simulink model "lab3_5_6"  (R2018a)
settings: Solver=VariableStepAuto  StartTime=0.0  StopTime=Tsim*Ts  RelTol=1e-3
values from neighbouring files (symbols this model uses):
  alpha = 0.99    [lab3.m]
  c_ik_init = zeros(26,1)    [lab3.m]
  coefHybrid = [0 0.2 1 0.3 -0.4 -0.1 0.1 -0.05 -0.02 -0.01]    [lab3.m]
  G = 0.1    [lab3.m]
  mu = mu_try(i)    [lab3.m]
  scramblerLocal = [3 5]    [lab3.m]
  scramblerRemote = [5 7]    [lab3.m]
  Ts = 1    [lab3.m]
settings Model: Creator=leonardopedroso  LastModifiedBy=leonardopedroso

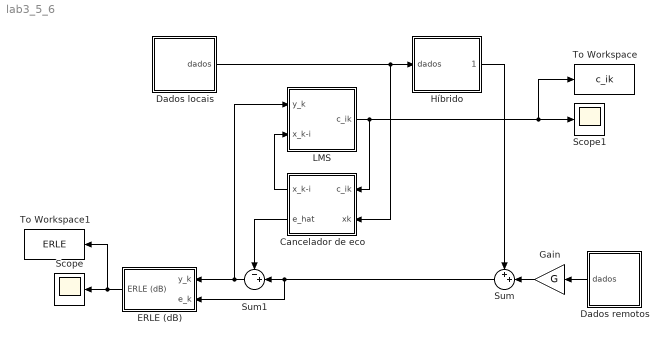
== system lab3_5_6 ==
  "Cancelador de eco " : Subsystem
  Dados locais : Subsystem
  Dados remotos : Subsystem
  ERLE (dB) : Subsystem
  Gain : Gain  Gain=G
  Híbrido : Subsystem
  LMS : Subsystem
  Scope : Scope
  Scope1 : Scope
  Sum : Sum  Inputs=++|
  Sum1 : Sum  Inputs=-+|
  To Workspace : ToWorkspace  VariableName=c_ik  SaveFormat=Timeseries  SampleTime=-1
  To Workspace1 : ToWorkspace  VariableName=ERLE  SaveFormat=Timeseries  SampleTime=-1
  wires:
  Dados locais/1(dados) -> Híbrido/1(dados), "Cancelador de eco "/2("xk ")
  Híbrido/1(híbrido) -> Sum/1
  Gain/1 -> Sum/2
  Dados remotos/1(dados) -> Gain/1
  Sum/1 -> Sum1/2, ERLE (dB)/2(e_k)
  LMS/1(c_ik) -> "Cancelador de eco "/1(c_ik), Scope1/1, To Workspace/1
  Sum1/1 -> ERLE (dB)/1(y_k), LMS/1("y_k ")
  "Cancelador de eco "/2("e_hat ") -> Sum1/1
  "Cancelador de eco "/1(x_k-i) -> LMS/2(x_k-i)
  ERLE (dB)/1(ERLE (dB)) -> To Workspace1/1, Scope/1

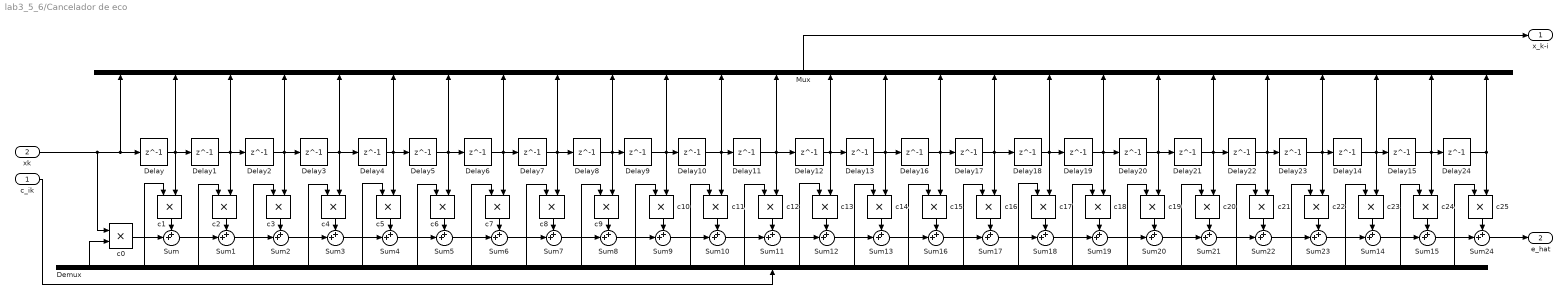
== system lab3_5_6/Cancelador de eco  ==
  c_ik : Inport
  "xk " : Inport  Port=2
  Delay{,1..24} (25 alike) : Delay  DelayLength=1  SampleTime=Ts
  Demux : Demux  Outputs=26
  Mux : Mux  Inputs=26
  Sum{,1..24} (25 alike) : Sum  Inputs=++|
  c{0..25} (26 alike) : Product
  x_k-i : Outport
  "e_hat " : Outport  Port=2
  wires:
  "xk "/1 -> Delay/1, Mux/1, c0/1
  Delay/1 -> Delay1/1, Mux/2, c1/2
  Delay1/1 -> Delay2/1, Mux/3, c2/2
  Delay2/1 -> Mux/4, Delay3/1, c3/2
  c1/1 -> Sum/1
  c0/1 -> Sum/2
  c3/1 -> Sum2/1
  c2/1 -> Sum1/1
  c4/1 -> Sum3/1
  Sum/1 -> Sum1/2
  Sum1/1 -> Sum2/2
  Sum2/1 -> Sum3/2
  c_ik/1 -> Demux/1
  Demux/5 -> c4/1
  Demux/4 -> c3/1
  Demux/3 -> c2/1
  Demux/2 -> c1/1
  Demux/1 -> c0/2
  c7/1 -> Sum6/1
  Delay5/1 -> Delay6/1, Mux/7, c6/2
  Delay4/1 -> Delay5/1, Mux/6, c5/2
  c8/1 -> Sum7/1
  Sum5/1 -> Sum6/2
  Sum4/1 -> Sum5/2
  Sum6/1 -> Sum7/2
  c6/1 -> Sum5/1
  Demux/8 -> c7/1
  Sum3/1 -> Sum4/2
  c5/1 -> Sum4/1
  Demux/6 -> c5/1
  Demux/7 -> c6/1
  Demux/9 -> c8/1
  Delay6/1 -> Mux/8, Delay7/1, c7/2
  Delay3/1 -> Mux/5, Delay4/1, c4/2
  c11/1 -> Sum10/1
  Delay9/1 -> c10/2, Mux/11, Delay10/1
  Delay8/1 -> c9/2, Mux/10, Delay9/1
  c12/1 -> Sum11/1
  Sum9/1 -> Sum10/2
  Sum8/1 -> Sum9/2
  Sum10/1 -> Sum11/2
  c10/1 -> Sum9/1
  Demux/12 -> c11/1
  Sum7/1 -> Sum8/2
  c9/1 -> Sum8/1
  Demux/10 -> c9/1
  Demux/11 -> c10/1
  Demux/13 -> c12/1
  Delay10/1 -> c11/2, Delay11/1, Mux/12
  Delay7/1 -> Mux/9, Delay8/1, c8/2
  Sum21/1 -> Sum22/2
  Demux/19 -> c18/1
  Delay12/1 -> Mux/14, Delay13/1, c13/2
  c15/1 -> Sum16/1
  c24/1 -> Sum15/1
  Demux/25 -> c24/1
  Demux/22 -> c21/1
  Demux/23 -> c22/1
  Sum16/1 -> Sum17/2
  Delay22/1 -> Mux/22, c21/2, Delay23/1
  c21/1 -> Sum22/1
  Demux/20 -> c19/1
  c22/1 -> Sum23/1
  c16/1 -> Sum17/1
  Delay13/1 -> Mux/15, Delay16/1, c14/2
  c18/1 -> Sum19/1
  Sum13/1 -> Sum16/2
  Sum12/1 -> Sum13/2
  Demux/15 -> c14/1
  Delay17/1 -> Mux/17, Delay18/1, c16/2
  Delay11/1 -> Delay12/1, Mux/13, c12/2
  Demux/16 -> c15/1
  Sum11/1 -> Sum12/2
  c14/1 -> Sum13/1
  c13/1 -> Sum12/1
  Demux/17 -> c16/1
  Demux/14 -> c13/1
  Demux/24 -> c23/1
  Sum22/1 -> Sum23/2
  Sum17/1 -> Sum18/2
  Delay16/1 -> Mux/16, Delay17/1, c15/2
  Demux/18 -> c17/1
  Delay18/1 -> Mux/18, Delay19/1, c17/2
  c19/1 -> Sum20/1
  Demux/21 -> c20/1
  Delay20/1 -> Mux/20, Delay21/1, c19/2
  Delay19/1 -> Mux/19, Delay20/1, c18/2
  Sum19/1 -> Sum20/2
  c20/1 -> Sum21/1
  c17/1 -> Sum18/1
  Sum18/1 -> Sum19/2
  Sum20/1 -> Sum21/2
  Delay21/1 -> Mux/21, Delay22/1, c20/2
  Sum14/1 -> Sum15/2
  Sum23/1 -> Sum14/2
  Delay23/1 -> Mux/23, c22/2, Delay14/1
  c23/1 -> Sum14/1
  Delay14/1 -> Mux/24, c23/2, Delay15/1
  Delay15/1 -> Delay24/1, Mux/25, c24/2
  Delay24/1 -> Mux/26, c25/2
  Sum15/1 -> Sum24/2
  c25/1 -> Sum24/1
  Demux/26 -> c25/1
  Sum24/1 -> "e_hat "/1
  Mux/1 -> x_k-i/1

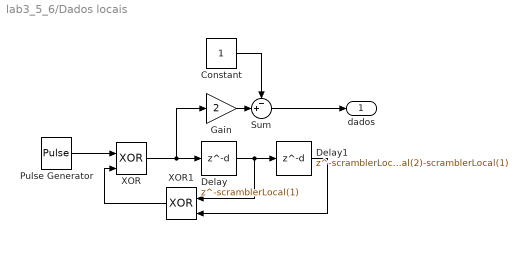
== system lab3_5_6/Dados locais ==
  Constant : Constant
  Delay : Delay  DelayLength=scramblerLocal(1)  SampleTime=Ts
  Delay1 : Delay  DelayLength=scramblerLocal(2)-scramblerLocal(1)  SampleTime=Ts
  Gain : Gain  Gain=2
  Pulse Generator : DiscretePulseGenerator  PulseType=Time based  Period=2*Ts  PulseWidth=50
  Sum : Sum  Inputs=-+|
  XOR : Logic  Operator=XOR  IconShape=distinctive  AllPortsSameDT=off  OutDataTypeStr=boolean
  XOR1 : Logic  Operator=XOR  IconShape=distinctive  AllPortsSameDT=off  OutDataTypeStr=boolean
  dados : Outport
  wires:
  Pulse Generator/1 -> XOR/1
  XOR1/1 -> XOR/2
  Delay/1 -> XOR1/1, Delay1/1
  Delay1/1 -> XOR1/2
  Gain/1 -> Sum/2
  Constant/1 -> Sum/1
  XOR/1 -> Delay/1, Gain/1
  Sum/1 -> dados/1

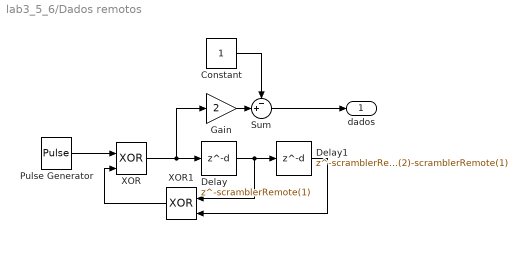
== system lab3_5_6/Dados remotos ==
  Constant : Constant
  Delay : Delay  DelayLength=scramblerRemote(1)  SampleTime=Ts
  Delay1 : Delay  DelayLength=scramblerRemote(2)-scramblerRemote(1)  SampleTime=Ts
  Gain : Gain  Gain=2
  Pulse Generator : DiscretePulseGenerator  PulseType=Time based  Period=2*Ts  PulseWidth=50
  Sum : Sum  Inputs=-+|
  XOR : Logic  Operator=XOR  IconShape=distinctive  AllPortsSameDT=off  OutDataTypeStr=boolean
  XOR1 : Logic  Operator=XOR  IconShape=distinctive  AllPortsSameDT=off  OutDataTypeStr=boolean
  dados : Outport
  wires:
  Pulse Generator/1 -> XOR/1
  XOR1/1 -> XOR/2
  Delay/1 -> XOR1/1, Delay1/1
  Delay1/1 -> XOR1/2
  Gain/1 -> Sum/2
  Constant/1 -> Sum/1
  XOR/1 -> Delay/1, Gain/1
  Sum/1 -> dados/1

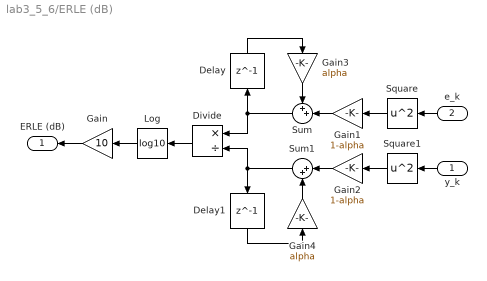
== system lab3_5_6/ERLE (dB) ==
  y_k : Inport
  e_k : Inport  Port=2
  Delay : Delay  DelayLength=1  SampleTime=Ts
  Delay1 : Delay  DelayLength=1  SampleTime=Ts
  Divide : Product  Inputs=*/
  Gain : Gain  Gain=10
  Gain1 : Gain  Gain=1-alpha
  Gain2 : Gain  Gain=1-alpha
  Gain3 : Gain  Gain=alpha
  Gain4 : Gain  Gain=alpha
  Log : Math  Operator=log10  SaturateOnIntegerOverflow=on
  Square : Math  Operator=square  SaturateOnIntegerOverflow=on
  Square1 : Math  Operator=square  SaturateOnIntegerOverflow=on
  Sum : Sum  Inputs=++|
  Sum1 : Sum  Inputs=|++
  ERLE (dB) : Outport
  wires:
  Gain/1 -> ERLE (dB)/1
  Log/1 -> Gain/1
  Divide/1 -> Log/1
  e_k/1 -> Square/1
  y_k/1 -> Square1/1
  Square/1 -> Gain1/1
  Square1/1 -> Gain2/1
  Gain1/1 -> Sum/2
  Sum/1 -> Divide/1, Delay/1
  Delay/1 -> Gain3/1
  Gain3/1 -> Sum/1
  Delay1/1 -> Gain4/1
  Sum1/1 -> Divide/2, Delay1/1
  Gain2/1 -> Sum1/1
  Gain4/1 -> Sum1/2

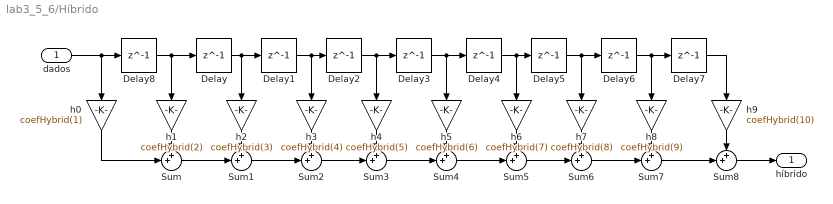
== system lab3_5_6/Híbrido ==
  dados : Inport
  Delay{,1..8} (9 alike) : Delay  DelayLength=1  SampleTime=Ts
  Sum{,1..8} (9 alike) : Sum  Inputs=++|
  h0 : Gain  Gain=coefHybrid(1)
  h1 : Gain  Gain=coefHybrid(2)
  h2 : Gain  Gain=coefHybrid(3)
  h3 : Gain  Gain=coefHybrid(4)
  h4 : Gain  Gain=coefHybrid(5)
  h5 : Gain  Gain=coefHybrid(6)
  h6 : Gain  Gain=coefHybrid(7)
  h7 : Gain  Gain=coefHybrid(8)
  h8 : Gain  Gain=coefHybrid(9)
  h9 : Gain  Gain=coefHybrid(10)
  híbrido : Outport
  wires:
  dados/1 -> h0/1, Delay8/1
  Delay/1 -> h2/1, Delay1/1
  Delay1/1 -> h3/1, Delay2/1
  Delay2/1 -> Delay3/1, h4/1
  Delay3/1 -> h5/1, Delay4/1
  Delay4/1 -> h6/1, Delay5/1
  Delay6/1 -> Delay7/1, h8/1
  Delay5/1 -> Delay6/1, h7/1
  Delay7/1 -> h9/1
  h0/1 -> Sum/2
  Delay8/1 -> h1/1, Delay/1
  h1/1 -> Sum/1
  Sum8/1 -> híbrido/1
  Sum/1 -> Sum1/2
  h2/1 -> Sum1/1
  h3/1 -> Sum2/1
  Sum1/1 -> Sum2/2
  h4/1 -> Sum3/1
  Sum2/1 -> Sum3/2
  h5/1 -> Sum4/1
  Sum3/1 -> Sum4/2
  h6/1 -> Sum5/1
  Sum4/1 -> Sum5/2
  Sum5/1 -> Sum6/2
  h7/1 -> Sum6/1
  h8/1 -> Sum7/1
  h9/1 -> Sum8/1
  Sum7/1 -> Sum8/2
  Sum6/1 -> Sum7/2

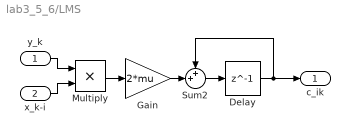
== system lab3_5_6/LMS ==
  "y_k " : Inport
  x_k-i : Inport  Port=2
  Delay : Delay  DelayLength=1  InitialCondition=c_ik_init  SampleTime=Ts
  Gain : Gain  Gain=2*mu
  Multiply : Product
  Sum2 : Sum  Inputs=++|
  c_ik : Outport
  wires:
  Delay/1 -> c_ik/1, Sum2/1
  Gain/1 -> Sum2/2
  Sum2/1 -> Delay/1
  Multiply/1 -> Gain/1
  x_k-i/1 -> Multiply/2
  "y_k "/1 -> Multiply/1
